simulink model "compswitchA"  (R2023a)
settings: Solver=VariableStepAuto  StartTime=0.0  StopTime=10.0  RelTol=1e-3
libraries: NSA_DEVS_SINKS x4, NSA_DEVS_MATH_OPERATIONS x2, NSA_DEVS_LOGISTICS x2, NSA_DEVS_ROUTING x1, NSA_DEVS_SOURCES x1
settings Model: Creator=peter  LastModifiedBy=david

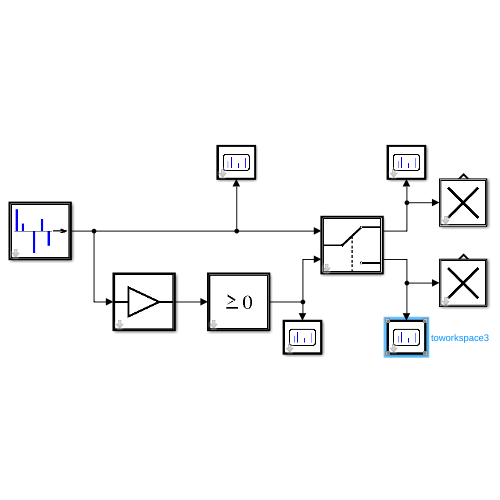
[thumbnail: Simulink's stored preview of the top-level diagram]
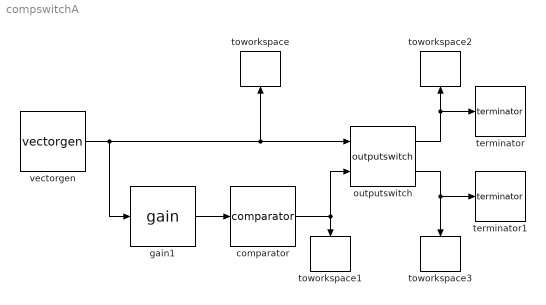
== system compswitchA ==
  comparator : NSA_DEVS_MATH_OPERATIONS/comparator  tau=[0,1]  debug=0
  gain1 : NSA_DEVS_MATH_OPERATIONS/gain  g=1  tau=[0,1]  debug=0
  outputswitch : NSA_DEVS_ROUTING/outputswitch  port0=1  tau=[0,2]  debug=0
  terminator : NSA_DEVS_LOGISTICS/terminator  tau=[0,1]  debug=0
  terminator1 : NSA_DEVS_LOGISTICS/terminator  tau=[0,1]  debug=0
  toworkspace : NSA_DEVS_SINKS/toworkspace  varname="\"vgenOut\""  t0=0  format="\"vector\""  tau=[0,5]  debug=0
  toworkspace1 : NSA_DEVS_SINKS/toworkspace  varname="\"compOut\""  t0=0  format="\"vector\""  tau=[0,5]  debug=0
  toworkspace2 : NSA_DEVS_SINKS/toworkspace  varname="\"sw1Out\""  t0=0  format="\"vector\""  tau=[0,5]  debug=0
  toworkspace3 : NSA_DEVS_SINKS/toworkspace  varname="\"sw2Out\""  t0=0  format="\"vector\""  tau=[0,5]  debug=0
  vectorgen : NSA_DEVS_SOURCES/vectorgen  tvec=[1, 3, 7, 8, 9]  yvec=[2, -3, -2, 1, -1]  tau=[0,1]  debug=0
  wires:
  vectorgen/1 -> gain1/1, toworkspace/1, outputswitch/1
  outputswitch/1 -> terminator/1, toworkspace2/1
  outputswitch/2 -> terminator1/1, toworkspace3/1
  comparator/1 -> toworkspace1/1, outputswitch/2
  gain1/1 -> comparator/1
